simulink model "adpative"  (R2016a)
settings: Solver=VariableStepAuto  StartTime=0.0  StopTime=10.0  RelTol=1e-3
settings Model: Creator=Aniket  LastModifiedBy=Aniket

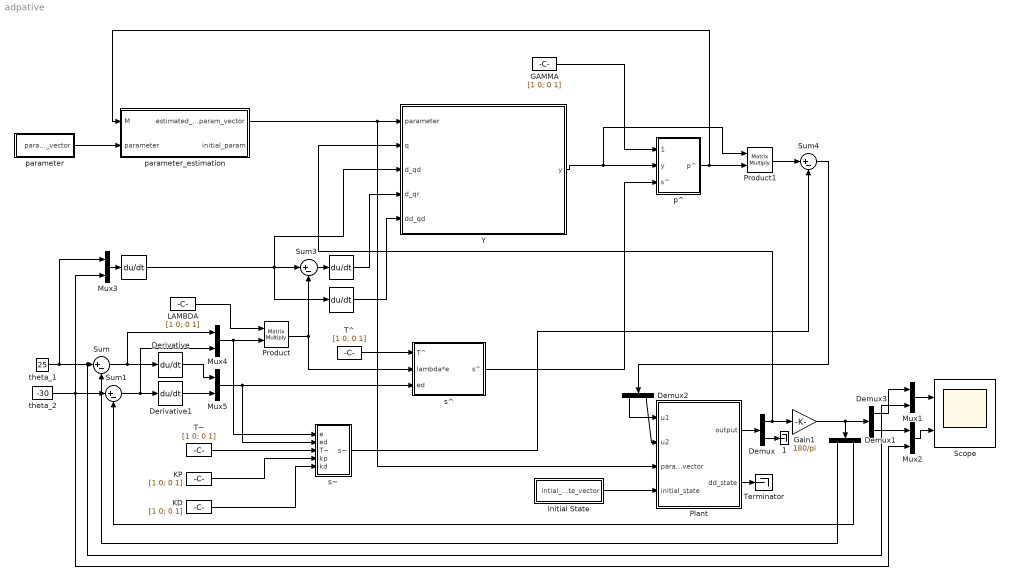
== system adpative ==
  "      " : Derivative
  "                 " : Derivative
  "                       " : Derivative
  "  1" : Terminator
  "  T^" : Constant  Value=[1 0; 0 1]
  "  T~" : Constant  Value=[1 0; 0 1]
  Demux{,1..3} (4 alike) : Demux  Outputs=2
  Derivative : Derivative
  Derivative1 : Derivative
  GAMMA : Constant  Value=[1 0; 0 1]
  Gain1 : Gain  Gain=180/pi
  Initial State : Subsystem
  KD : Constant  Value=[1 0; 0 1]
  KP : Constant  Value=[1 0; 0 1]
  LAMBDA : Constant  Value=[1 0; 0 1]
  Mux{1..5} (5 alike) : Mux  Inputs=2
  Plant : Subsystem
  Product : Product  Multiplication=Matrix(*)
  Product1 : Product  Multiplication=Matrix(*)
  Scope : Scope  NumInputPorts=2
  Sum{,1,3..4} (4 alike) : Sum  Inputs=|+-
  Terminator : Terminator
  Y : MATLAB Function  TreatAsAtomicUnit=on
  p^ : Subsystem
  parameter : Subsystem
  parameter_estimation : Subsystem
  s^ : Subsystem
  s~ : Subsystem
  theta_1 : Constant  Value=25
  theta_2 : Constant  Value=-30
  wires:
  Plant/2(dd_state) -> Terminator/1
  Initial State/1(intial_state_vector) -> Plant/4(initial_state)
  Demux/1 -> Y/2(q), Gain1/1
  Gain1/1 -> Demux3/1, Demux1/1
  Demux1/1 -> Sum/2
  Demux1/2 -> Sum1/2
  Demux/2 -> "  1"/1
  Plant/1(output) -> Demux/1
  theta_1/1 -> Mux3/1, Sum/1, Mux1/2
  theta_2/1 -> Mux3/2, Mux2/2, Sum1/1
  Sum/1 -> Mux4/1, Derivative/1
  Sum1/1 -> Mux4/2, Derivative1/1
  Derivative1/1 -> Mux5/2
  Derivative/1 -> Mux5/1
  Demux2/1 -> Plant/1(u1)
  Demux2/2 -> Plant/2(u2)
  Mux1/1 -> Scope/1
  Demux3/1 -> Mux1/1
  Demux3/2 -> Mux2/1
  Mux2/1 -> Scope/2
  Mux3/1 -> "      "/1
  "      "/1 -> "                       "/1, Y/3(d_qd), Sum3/1
  LAMBDA/1 -> Product/1
  Product/1 -> s^/2(lambda*e), Sum3/2
  Mux4/1 -> s~/1(e), Product/2
  Sum3/1 -> "                 "/1
  "                 "/1 -> Y/4(d_qr)
  "                       "/1 -> Y/5(dd_qd)
  "  T^"/1 -> s^/1(T^)
  Mux5/1 -> s~/2(ed), s^/3(ed)
  GAMMA/1 -> p^/1(GAMMA)
  Y/1(y) -> Product1/1, p^/2(y)
  s^/1(s^) -> p^/3(s^)
  Product1/1 -> Sum4/1
  Sum4/1 -> Demux2/1
  "  T~"/1 -> s~/3(T~)
  KP/1 -> s~/4(kp)
  KD/1 -> s~/5(kd)
  s~/1(s~) -> Sum4/2
  p^/1(p^) -> Product1/2, parameter_estimation/1(M)
  parameter/1("param_vector ") -> parameter_estimation/2(parameter)
  parameter_estimation/1(estimated_param_vector) -> Y/1(parameter), Plant/3(param_vector)

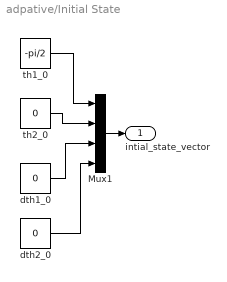
== system adpative/Initial State ==
  Mux1 : Mux
  dth1_0 : Constant  Value=0
  dth2_0 : Constant  Value=0
  th1_0 : Constant  Value=-pi/2
  th2_0 : Constant  Value=0
  intial_state_vector : Outport
  wires:
  Mux1/1 -> intial_state_vector/1
  dth2_0/1 -> Mux1/4
  th1_0/1 -> Mux1/1
  dth1_0/1 -> Mux1/3
  th2_0/1 -> Mux1/2

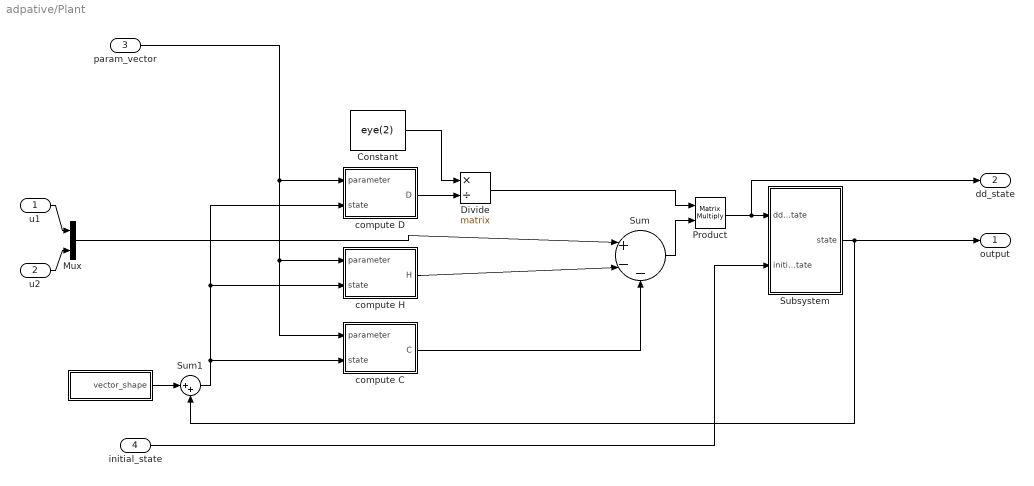
== system adpative/Plant ==
  u1 : Inport
  u2 : Inport  Port=2
  param_vector : Inport  Port=3
  initial_state : Inport  Port=4
  "  " : Subsystem
  Constant : Constant  Value=eye(2)
  Divide : Product  Inputs=*/  Multiplication=Matrix(*)
  Mux : Mux  Inputs=2
  Product : Product  Multiplication=Matrix(*)
  Subsystem : Subsystem
  Sum : Sum  Inputs=|+--
  Sum1 : Sum  Inputs=|++
  compute C : MATLAB Function  TreatAsAtomicUnit=on
  compute D : MATLAB Function  TreatAsAtomicUnit=on
  compute H : MATLAB Function  TreatAsAtomicUnit=on
  output : Outport
  dd_state : Outport  Port=2
  wires:
  Sum/1 -> Product/2
  compute C/1(C) -> Sum/3
  Constant/1 -> Divide/1
  initial_state/1 -> Subsystem/2(initial_state)
  compute H/1(H) -> Sum/2
  compute D/1(D) -> Divide/2
  Mux/1 -> Sum/1
  param_vector/1 -> compute C/1(parameter), compute H/1(parameter), compute D/1(parameter)
  Product/1 -> dd_state/1, Subsystem/1(dd_state)
  Sum1/1 -> compute D/2(state), compute H/2(state), compute C/2(state)
  "  "/1(vector_shape) -> Sum1/1
  Divide/1 -> Product/1
  u1/1 -> Mux/1
  Subsystem/1(state) -> output/1, Sum1/2
  u2/1 -> Mux/2

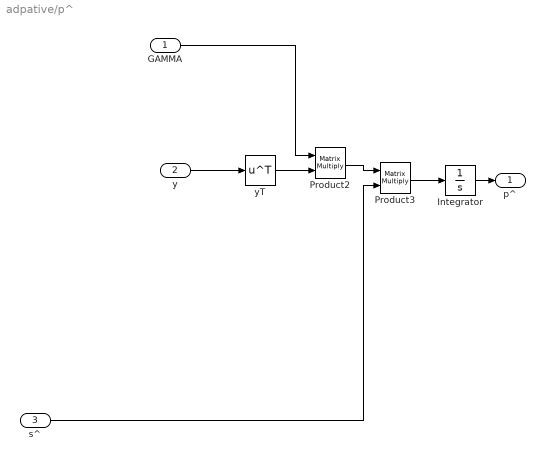
== system adpative/p^ ==
  GAMMA : Inport
  y : Inport  Port=2
  s^ : Inport  Port=3
  Integrator : Integrator
  Product2 : Product  Multiplication=Matrix(*)
  Product3 : Product  Multiplication=Matrix(*)
  yT : Math  Operator=transpose  SaturateOnIntegerOverflow=on
  p^ : Outport
  wires:
  Integrator/1 -> p^/1
  yT/1 -> Product2/2
  GAMMA/1 -> Product2/1
  s^/1 -> Product3/2
  Product2/1 -> Product3/1
  y/1 -> yT/1
  Product3/1 -> Integrator/1

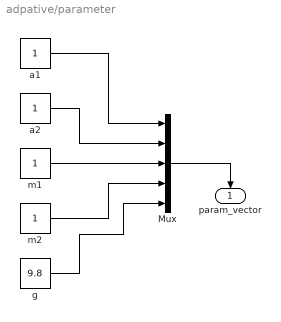
== system adpative/parameter ==
  Mux : Mux  Inputs=5
  "a1 " : Constant
  a2 : Constant
  g : Constant  Value=9.8
  m1 : Constant
  m2 : Constant
  "param_vector " : Outport
  wires:
  m1/1 -> Mux/3
  Mux/1 -> "param_vector "/1
  g/1 -> Mux/5
  "a1 "/1 -> Mux/1
  m2/1 -> Mux/4
  a2/1 -> Mux/2

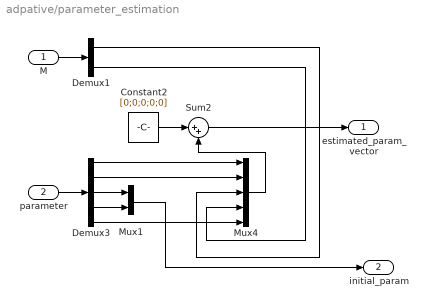
== system adpative/parameter_estimation ==
  M : Inport
  parameter : Inport  Port=2
  Constant2 : Constant  Value=[0;0;0;0;0]
  Demux1 : Demux  Outputs=2
  Demux3 : Demux  Outputs=5
  Mux1 : Mux  Inputs=2
  Mux4 : Mux  Inputs=5
  Sum2 : Sum  Inputs=|++
  estimated_param_vector : Outport
  initial_param : Outport  Port=2
  wires:
  Demux1/1 -> Mux4/3
  Demux3/4 -> Mux1/2
  Demux3/3 -> Mux1/1
  Mux4/1 -> Sum2/2
  Demux3/5 -> Mux4/5
  Demux1/2 -> Mux4/4
  Demux3/1 -> Mux4/1
  Demux3/2 -> Mux4/2
  parameter/1 -> Demux3/1
  Sum2/1 -> estimated_param_vector/1
  Constant2/1 -> Sum2/1
  Mux1/1 -> initial_param/1
  M/1 -> Demux1/1

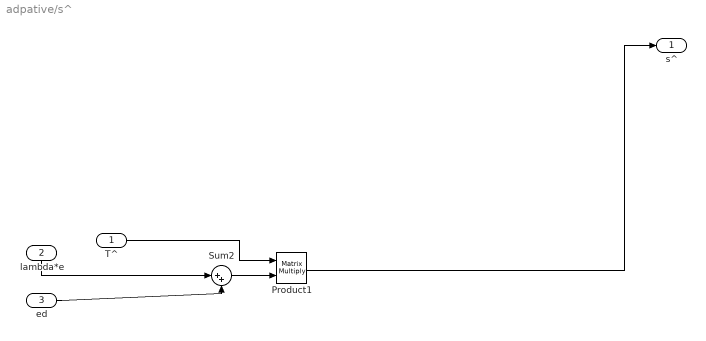
== system adpative/s^ ==
  T^ : Inport
  lambda*e : Inport  Port=2
  ed : Inport  Port=3
  Product1 : Product  Multiplication=Matrix(*)
  Sum2 : Sum  Inputs=|++
  s^ : Outport
  wires:
  T^/1 -> Product1/1
  Sum2/1 -> Product1/2
  lambda*e/1 -> Sum2/1
  Product1/1 -> s^/1
  ed/1 -> Sum2/2

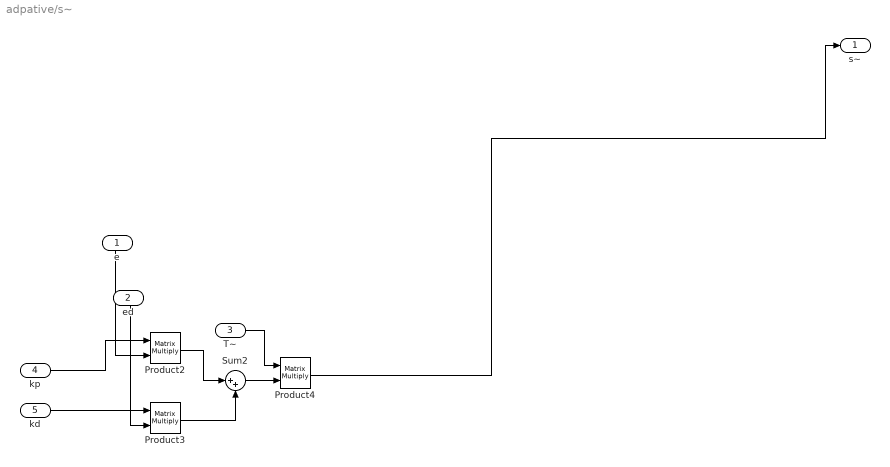
== system adpative/s~ ==
  e : Inport
  ed : Inport  Port=2
  T~ : Inport  Port=3
  kp : Inport  Port=4
  kd : Inport  Port=5
  Product2 : Product  Multiplication=Matrix(*)
  Product3 : Product  Multiplication=Matrix(*)
  Product4 : Product  Multiplication=Matrix(*)
  Sum2 : Sum  Inputs=|++
  s~ : Outport
  wires:
  kd/1 -> Product3/1
  Product3/1 -> Sum2/2
  Product4/1 -> s~/1
  T~/1 -> Product4/1
  Product2/1 -> Sum2/1
  Sum2/1 -> Product4/2
  ed/1 -> Product3/2
  kp/1 -> Product2/1
  e/1 -> Product2/2

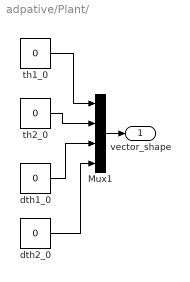
== system adpative/Plant/   ==
  Mux1 : Mux
  dth1_0 : Constant  Value=0
  dth2_0 : Constant  Value=0
  th1_0 : Constant  Value=0
  th2_0 : Constant  Value=0
  vector_shape : Outport
  wires:
  th2_0/1 -> Mux1/2
  dth1_0/1 -> Mux1/3
  th1_0/1 -> Mux1/1
  dth2_0/1 -> Mux1/4
  Mux1/1 -> vector_shape/1

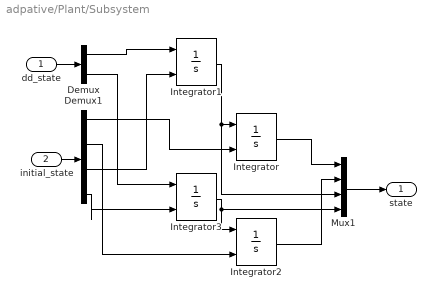
== system adpative/Plant/Subsystem ==
  dd_state : Inport
  initial_state : Inport  Port=2
  Demux : Demux  Outputs=2
  Demux1 : Demux
  Integrator{,1..3} (4 alike) : Integrator  InitialConditionSource=external
  Mux1 : Mux
  state : Outport
  wires:
  initial_state/1 -> Demux1/1
  dd_state/1 -> Demux/1
  Integrator/1 -> Mux1/1
  Integrator2/1 -> Mux1/2
  Demux/1 -> Integrator1/1
  Demux/2 -> Integrator3/1
  Integrator1/1 -> Mux1/3, Integrator/1
  Integrator3/1 -> Mux1/4, Integrator2/1
  Demux1/3 -> Integrator1/2
  Demux1/4 -> Integrator3/2
  Mux1/1 -> state/1
  Demux1/2 -> Integrator2/2
  Demux1/1 -> Integrator/2

== matlab function adpative/Plant/compute D ==
  data: parameter input; D output; state input
function D = D(parameter,state)
a1 = parameter(1);
a2 = parameter(2);
m1 = parameter(3);
m2 = parameter(4);
g = parameter(5);

if isempty(state)
    th1 = 0;
    th2 = 0;
    thd1 = 0;
    thd2 = 0;
else
    th1 = state(1);
    th2 = state(2);
    thd1 = state(3);
    thd2 = state(4);
end

D = [ (a1^2*m1)/3 + a1^2*m2 + (a2^2*m2)/3 + a1*a2*m2*cos(th2), (a2*m2*(2*a2 + 3*a1*cos(th2)))/6;
    (a2*m2*(2*a2 + 3*a1*cos(th2)))/6,                      (a2^2*m2)/3];

== matlab function adpative/Y ==
  data: parameter input; y output; q input; d_qd input; d_qr input; dd_qd input
function y = Y(parameter,q,d_qd,d_qr,dd_qd)
a1 = parameter(1);
a2 = parameter(2);
m1 = parameter(3);
m2 = parameter(4);
g = parameter(5);
th1 = q(1);
th2 = q(2);
thd1 = d_qr(1);
thd2 = d_qr(2);
qdd1 = dd_qd(1);
qdd2 = dd_qd(2);
y = [((qdd1*a1^2)/3 + (g*cos(th1)*a1)/2), (qdd1*(a1^2 + cos(th2)*a1*a2 + a2^2/3) + (g*(a2*cos(th1 + th2) + 2*a1*cos(th1)))/2 + (a2*qdd2*(2*a2 + 3*a1*cos(th2)))/6 - (a1*a2*thd2*sin(th2)*(2*thd1 + thd2))/2);
                                  0,                                                        ((a2^2*qdd2)/3 + (a2*g*cos(th1 + th2))/2 + (a2*qdd1*(2*a2 + 3*a1*cos(th2)))/6 + (a1*a2*thd1^2*sin(th2))/2)];

== matlab function adpative/Plant/compute C ==
  data: parameter input; C output; state input
function C = C(parameter,state)
a1 = parameter(1);
a2 = parameter(2);
m1 = parameter(3);
m2 = parameter(4);
g = parameter(5);
if isempty(state)
    th1 = 0;
    th2 = 0;
    thd1 = 0;
    thd2 = 0;
else
    th1 = state(1);
    th2 = state(2);
    thd1 = state(3);
    thd2 = state(4);
end
C = [(g*(a1*m1*cos(th1) + 2*a1*m2*cos(th1) + a2*m2*cos(th1 + th2)))/2;
                                       (a2*g*m2*cos(th1 + th2))/2];

== matlab function adpative/Plant/compute H ==
  data: parameter input; H output; state input
function H = H(parameter,state)
a1 = parameter(1);
a2 = parameter(2);
m1 = parameter(3);
m2 = parameter(4);
g = parameter(5);

if isempty(state)
    th1 = 0;
    th2 = 0;
    thd1 = 0;
    thd2 = 0;
else
    th1 = state(1);
    th2 = state(2);
    thd1 = state(3);
    thd2 = state(4);
end
H = [ -(a1*a2*m2*thd2*sin(th2)*(2*thd1 + thd2))/2;
                (a1*a2*m2*thd1^2*sin(th2))/2];
